simulink model "Sim_Plant_z"  (R2017a)
settings: Solver=ode3  StartTime=0.0  StopTime=5  FixedStep=1/50  RelTol=1e-3  EnableMultiTasking=on
values from neighbouring files (symbols this model uses):
  mQ = 0.5645    [LG_ID_ss_Model.m]
undefined symbols (not defined in the file or in its folder): Kd_z, Kp_z
settings Model: Creator=GeoLee  LastModifiedBy=gmh_n
settings DataIOCC: LimitDataPoints=on  SaveFormat=Array
settings OptimizationCC: ExpressionDepthLimit=2147483647  LifeSpan=inf
settings DebuggingCC: UnderspecifiedInitializationDetection=Classic  MergeDetectMultiDrivingBlocksExec=none  SolverPrmCheckMsg=warning  StateNameClashWarn=warning  SFUnexpectedBacktrackingDiag=warning  SFNoUnconditionalDefaultTransitionDiag=warning  SFExecutionAtInitializationDiag=none
settings HardwareCC: ProdBitPerPointer=32  ProdBitPerSizeT=32  ProdBitPerPtrDiffT=32  ProdLargestAtomicFloat=None  ProdIntDivRoundTo=Undefined  ProdEndianess=Unspecified  ProdWordSize=32  ProdHWDeviceType=32-bit Generic
settings ModelReferenceCC: PropagateSignalLabelsOutOfModel=off
settings GRTTargetCC: TargetLangStandard=C89/C90 (ANSI)  GeneratePreprocessorConditionals=Disable all
settings ConfigComp: CovMetricSettings=dw  CovHtmlReporting=on  CovSaveCumulativeToWorkspaceVar=on  CovSaveSingleToWorkspaceVar=on  CovExternalEMLEnable=off

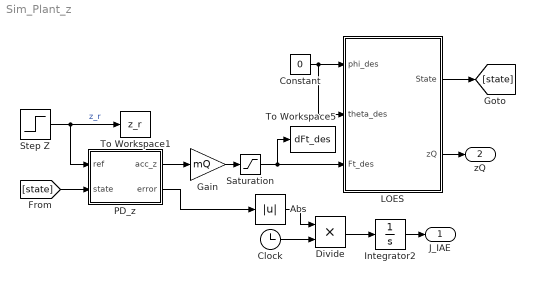
== system Sim_Plant_z ==
  Abs : Abs
  Clock : Clock
  Constant : Constant  Value=0
  Divide : Product  Inputs=**
  Gain : Gain  Gain=mQ
  Integrator2 : Integrator
  LOES : Subsystem
  PD_z : Subsystem
  Saturation : Saturate  UpperLimit=10  LowerLimit=-0.5645*9.8
  Step Z : Step  After=0.2  SampleTime=0
  To Workspace1 : ToWorkspace  VariableName=z_r  SampleTime=-1
  To Workspace5 : ToWorkspace  VariableName=dFt_des  SampleTime=-1
  J_IAE : Outport
  zQ : Outport  Port=2
  wires:
  LOES/1(State) -> [state]
  [state] -> PD_z/2(state)
  Step Z/1 -> PD_z/1(ref), To Workspace1/1  "z_r"
  PD_z/1(acc_z) -> Gain/1
  Saturation/1 -> To Workspace5/1, LOES/3(Ft_des)
  Integrator2/1 -> J_IAE/1
  Divide/1 -> Integrator2/1
  Clock/1 -> Divide/2
  Abs/1 -> Divide/1
  PD_z/2(error) -> Abs/1
  LOES/2(zQ) -> zQ/1
  Gain/1 -> Saturation/1
  Constant/1 -> LOES/2(theta_des), LOES/1(phi_des)

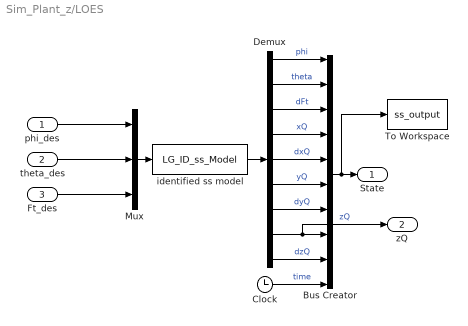
== system Sim_Plant_z/LOES ==
  phi_des : Inport
  theta_des : Inport  Port=2
  Ft_des : Inport  Port=3
  Bus Creator : BusCreator  Inputs=10
  Clock : Clock
  Demux : Demux  Outputs=9
  Mux : Mux  Inputs=3
  To Workspace : ToWorkspace  VariableName=ss_output  SampleTime=-1
  identified ss model : S-Function  FunctionName=LG_ID_ss_Model  SFunctionDeploymentMode=off  EnableBusSupport=off
  State : Outport
  zQ : Outport  Port=2
  wires:
  Clock/1 -> Bus Creator/10  "time"
  identified ss model/1 -> Demux/1
  Mux/1 -> identified ss model/1
  Ft_des/1 -> Mux/3
  phi_des/1 -> Mux/1
  theta_des/1 -> Mux/2
  Demux/6 -> Bus Creator/6  "yQ"
  Demux/7 -> Bus Creator/7  "dyQ"
  Demux/4 -> Bus Creator/4  "xQ"
  Demux/9 -> Bus Creator/9  "dzQ"
  Demux/5 -> Bus Creator/5  "dxQ"
  Demux/1 -> Bus Creator/1  "phi"
  Demux/3 -> Bus Creator/3  "dFt"
  Demux/2 -> Bus Creator/2  "theta"
  Demux/8 -> zQ/1, Bus Creator/8  "zQ"
  Bus Creator/1 -> To Workspace/1, State/1

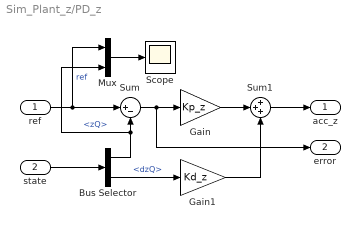
== system Sim_Plant_z/PD_z ==
  ref : Inport
  state : Inport  Port=2
  Bus Selector : BusSelector  OutputSignals=zQ,dzQ
  Gain : Gain  Gain=Kp_z
  Gain1 : Gain  Gain=Kd_z
  Mux : Mux  Inputs=2
  Scope : Scope
  Sum : Sum  Inputs=|+-
  Sum1 : Sum  Inputs=+++
  acc_z : Outport
  error : Outport  Port=2
  wires:
  Gain1/1 -> Sum1/3
  Sum1/1 -> acc_z/1
  Gain/1 -> Sum1/2
  Bus Selector/2 -> Gain1/1  "<dzQ>"
  state/1 -> Bus Selector/1
  Sum/1 -> Gain/1, error/1
  ref/1 -> Sum/1, Mux/1  "ref"
  Bus Selector/1 -> Mux/2, Sum/2  "<zQ>"
  Mux/1 -> Scope/1
